simulink library "SUB_ECU_L4_MABX_HW_Interface_PTC_1571"  (R2018a)
settings: Solver=VariableStepAuto  StartTime=0.0  StopTime=10.0  RelTol=1e-3
PostLoadFcn:
  | , if any(exist('dsrtsu_mdlpostloadfcn', 'file') == [2, 3, 6]), try dsrtsu_mdlpostloadfcn('Execute', bdroot); catch fprintf('Error in PostLoadFcn (dsrtsu_mdlpostloadfcn) for model "%s":\n %s\n', bdroot, lasterr); end, end,
undefined symbols (not defined in the file or in its folder): CANR_PROPB_REAX_3_13_CHANNEL_APV, CANR_PROPB_REAX_4_13_CHANNEL_APV, CANR_PROPB_XPR_1_50_CHANNEL_APV, ENUM_CAN_RX_T, ENUM_CAN_TX_T, ENUM_REAX_OPERATION_MODE_T, ENUM_SIGNAL_HEALTH_T, ENUM_XBR_CONTROL_MODE_T, ENUM_XBR_EBI_MODE_T, ENUM_XBR_PASS_THROUGH_ACTIVE_T, ENUM_XBR_PRIORITY_T, ENUM_XPR_INHIBIT_PARK_MANUAL_T, ENUM_XPR_INHIBIT_UNPARK_MANUAL_T, ENUM_XPR_PARK_MANUAL_T, ENUM_XPR_UNPARK_MANUAL_T, IGNITION_RELAY_OVERRIDE_APV, INVERTER_RELAY_OVERRIDE_APV, MABX_RELAY_OVERRIDE_APV, PROPB_REAX_1_E4_DES_POS_SIG_SRC_APV, PROPB_REAX_1_E4_DESIRED_OPMODE_APV, PROPB_REAX_1_E4_DESIRED_POSITION_APV, ptc_matlab_lib, SENSOR_RELAY_OVERRIDE_APV, sfi, sfp
libraries: PTC_MBDS_LIB x163, rtican x81, simulink x41, EmE_MBD_Blockset x35, rti1401lib_dio_type4 x8, simulink_need_slupdate x7, $bdroot x5, rti1401lib_adc_type4 x2, rti1401lib_aio_type1 x1, rtitasklib x1
(part 4 of 27)

== system SUB_ECU_L4_MABX_HW_Interface_PTC_1571/OUTPUTS_PTC_1571 ==
  Outputs : Inport
  In : Inport  Port=2
  CAN_Out_PTC_1571 : $bdroot/CAN_Out_PTC_1571
  DIGITAL_out : $bdroot/DIGITAL_out
  wires:
  In/1 -> DIGITAL_out/2, CAN_Out_PTC_1571/2
  Outputs/1 -> DIGITAL_out/1, CAN_Out_PTC_1571/1

== system SUB_ECU_L4_MABX_HW_Interface_PTC_1571/CAN_Out_PTC_1571/CAN_TX_10000ms ==
  10000msCAN : Inport
  Terminator : Terminator
  wires:
  10000msCAN/1 -> Terminator/1

== system SUB_ECU_L4_MABX_HW_Interface_PTC_1571/CAN_Out_PTC_1571/CAN_TX_1000ms ==
  1000msCAN : Inport
  CAN_TX_AIR1_31 : Subsystem
  CAN_TX_AMB_00 : Subsystem
  Constant1 : Constant  Value=ENUM_CAN_TX_T.TX_CAN_4
  Constant2 : Constant  Value=ENUM_CAN_TX_T.TX_CAN_4
  wires:
  Constant1/1 -> CAN_TX_AMB_00/1(Channel)
  1000msCAN/1 -> CAN_TX_AIR1_31/2(Data), CAN_TX_AMB_00/2(Data)
  Constant2/1 -> CAN_TX_AIR1_31/1(Channel)

== system SUB_ECU_L4_MABX_HW_Interface_PTC_1571/CAN_Out_PTC_1571/CAN_TX_100ms ==
  100msCAN : Inport
  Feedthrough : Inport  Port=2
  Bus Selector : BusSelector  OutputSignals=INPUTS.DIO_Bus.OperatorEnableSwitch,INPUTS.CAN.VI_00.F_Truck166_VIN_Match
  Bus Selector1 : BusSelector  OutputSignals=INPUTS.DIO_Bus.OperatorEnableSwitch
  Bus Selector2 : BusSelector  OutputSignals=INPUTS.DIO_Bus.OperatorEnableSwitch,INPUTS.CAN.VI_00.F_Truck1571_VIN_Match
  CANT_PROPB_XPR_5B_CHANNEL_APV : Constant  Value=ENUM_CAN_TX_T.TX_CAN_1
  CANT_PROPB_XPR_FC_CHANNEL_APV : Constant  Value=ENUM_CAN_TX_T.TX_CAN_4
  CAN_TX_CCVS1_00 : Subsystem
  CAN_TX_CCVS1_31 : Subsystem
  CAN_TX_EBC2_0B : Subsystem
  CAN_TX_ETC2_03 : Subsystem
  CAN_TX_PROPB_REAX_5_E4 : Subsystem
  CAN_TX_PROPB_XPR_5B : Subsystem
  CAN_TX_PROPB_XPR_FC : Subsystem
  COGSRapidUpdate : Subsystem
  EBC1_8B : Subsystem
  EffortsValue : Subsystem
  Encode_PropB_REAX_5 : Subsystem
  Encode_PropB_XPR_5B : Subsystem
  Encode_PropB_XPR_FC : Subsystem  SystemSampleTime=0.1
  Logical Operator : Logic  OutDataTypeStr=boolean
  Logical Operator1 : Logic  OutDataTypeStr=boolean
  POSRapidUpdate : Subsystem
  PROPB_XPR_INHIBIT_PARK_MANUAL_APV : Constant  Value=ENUM_XPR_INHIBIT_PARK_MANUAL_T.NO_OVERRIDE
  PROPB_XPR_INHIBIT_UNPARK_MANUAL_APV : Constant  Value=ENUM_XPR_INHIBIT_UNPARK_MANUAL_T.NO_OVERRIDE
  PROPB_XPR_PARK_MANUAL_APV : Constant  Value=ENUM_XPR_PARK_MANUAL_T.NO_OVERRIDE
  PROPB_XPR_UNPARK_MANUAL_APV : Constant  Value=ENUM_XPR_UNPARK_MANUAL_T.NO_OVERRIDE
  enableCOGSRapidUpdateTX : Constant  Value=boolean(1)
  enableEBC1_8B_TX : Constant  Value=boolean(1)
  enablePosRapidUpdateTX : Constant  Value=boolean(1)
  wires:
  Feedthrough/1 -> CAN_TX_PROPB_REAX_5_E4/1(enable), CAN_TX_CCVS1_00/1(Data), COGSRapidUpdate/2(Data), CAN_TX_CCVS1_31/1(Data), CAN_TX_ETC2_03/1(Data), CAN_TX_EBC2_0B/1(Data), EBC1_8B/2(Data)
  Logical Operator1/1 -> CAN_TX_PROPB_XPR_FC/1(Enable)
  Bus Selector2/2 -> Logical Operator1/2  "<F_Truck1571_VIN_Match>"
  Bus Selector2/1 -> Logical Operator1/1  "<OperatorEnableSwitch>"
  Bus Selector/2 -> Logical Operator/2  "<F_Truck166_VIN_Match>"
  Logical Operator/1 -> CAN_TX_PROPB_XPR_5B/1(Enable)
  Bus Selector/1 -> Logical Operator/1  "<OperatorEnableSwitch>"
  Encode_PropB_XPR_5B/1(Data) -> CAN_TX_PROPB_XPR_5B/3(RawData)
  CANT_PROPB_XPR_5B_CHANNEL_APV/1 -> CAN_TX_PROPB_XPR_5B/2(Channel)
  enableEBC1_8B_TX/1 -> EBC1_8B/1(Enable)
  Encode_PropB_REAX_5/1(Data) -> CAN_TX_PROPB_REAX_5_E4/2(RawData)
  EffortsValue/1(EffortsValue) -> Encode_PropB_REAX_5/1(EffortsValue)
  Bus Selector1/1 -> Encode_PropB_XPR_FC/5(F_MessageEnable)  "<OperatorEnableSwitch>"
  CANT_PROPB_XPR_FC_CHANNEL_APV/1 -> CAN_TX_PROPB_XPR_FC/2(Channel)
  Encode_PropB_XPR_FC/1(Data) -> CAN_TX_PROPB_XPR_FC/3(RawData)
  PROPB_XPR_INHIBIT_UNPARK_MANUAL_APV/1 -> Encode_PropB_XPR_5B/2(inhibit_unpark_manual), Encode_PropB_XPR_FC/2(inhibit_unpark_manual)
  PROPB_XPR_PARK_MANUAL_APV/1 -> Encode_PropB_XPR_5B/3(park_manual), Encode_PropB_XPR_FC/3(park_manual)
  PROPB_XPR_UNPARK_MANUAL_APV/1 -> Encode_PropB_XPR_5B/4(unpark_manual), Encode_PropB_XPR_FC/4(unpark_manual)
  PROPB_XPR_INHIBIT_PARK_MANUAL_APV/1 -> Encode_PropB_XPR_5B/1(inhibit_park_manual), Encode_PropB_XPR_FC/1(inhibit_park_manual)
  enableCOGSRapidUpdateTX/1 -> COGSRapidUpdate/1(Enable)
  enablePosRapidUpdateTX/1 -> POSRapidUpdate/1(Enable)
  100msCAN/1 -> Bus Selector/1, Bus Selector1/1, POSRapidUpdate/2(Data), Bus Selector2/1

== system SUB_ECU_L4_MABX_HW_Interface_PTC_1571/CAN_Out_PTC_1571/CAN_TX_10ms ==
  10msCAN : Inport
  In : Inport  Port=2
  CANT_ACCS_E4_CHANNEL_APV : Constant  Value=ENUM_CAN_TX_T.TX_CAN_4
  CANT_EEC1_00_CHANNEL_APV : Constant  Value=ENUM_CAN_TX_T.TX_CAN_4_5
  CANT_VDC2_0B_CHANNEL_APV : Constant  Value=ENUM_CAN_TX_T.TX_CAN_5
  CAN_TX_ACCS_E4 : Subsystem
  CAN_TX_EEC1_00 : Subsystem
  CAN_TX_PROPB_REAX_1_E4 : Subsystem
  CAN_TX_VDC2_0B : Subsystem
  Encode_PROPB_REAX_1 : Subsystem
  wires:
  In/1 -> CAN_TX_PROPB_REAX_1_E4/1(enable), CAN_TX_EEC1_00/2(Data)
  CANT_ACCS_E4_CHANNEL_APV/1 -> CAN_TX_ACCS_E4/1(Channel)
  CANT_EEC1_00_CHANNEL_APV/1 -> CAN_TX_EEC1_00/1(Channel)
  Encode_PROPB_REAX_1/1(Out1) -> CAN_TX_PROPB_REAX_1_E4/2(RawData)
  CANT_VDC2_0B_CHANNEL_APV/1 -> CAN_TX_VDC2_0B/1(Channel)
  10msCAN/1 -> CAN_TX_VDC2_0B/2(Data), CAN_TX_ACCS_E4/2(Data), Encode_PROPB_REAX_1/1(In1)

== system SUB_ECU_L4_MABX_HW_Interface_PTC_1571/CAN_Out_PTC_1571/CAN_TX_20ms ==
  20msCAN : Inport
  Bus Selector : BusSelector  OutputSignals=INPUTS.DIO_Bus.OperatorEnableSwitch
  CANT_PROPB_XBR_B3_CHANNEL_APV : Constant  Value=ENUM_CAN_TX_T.TX_DISABLED
  CANT_STD_ODOMETRY_CHANNEL_APV : Constant  Value=ENUM_CAN_TX_T.TX_CAN_6
  CAN_TX_PROPB_XBR_B3 : Subsystem
  CAN_TX_PropB_2C2_XPR_65 : Subsystem
  CAN_TX_STD_ODOMETRY : Subsystem
  Encode_PropB_2C2_XPR : Subsystem
  Encode_PropB_XBR_B3 : Subsystem
  wires:
  Bus Selector/1 -> CAN_TX_PROPB_XBR_B3/3(OperatorEnable)  "<OperatorEnableSwitch>"
  Encode_PropB_XBR_B3/1(Out) -> CAN_TX_PROPB_XBR_B3/2(Data)
  CANT_PROPB_XBR_B3_CHANNEL_APV/1 -> CAN_TX_PROPB_XBR_B3/1(Channel)
  CANT_STD_ODOMETRY_CHANNEL_APV/1 -> CAN_TX_STD_ODOMETRY/1(Channel)
  20msCAN/1 -> CAN_TX_STD_ODOMETRY/2(Data), Bus Selector/1, Encode_PropB_2C2_XPR/1(In), Encode_PropB_XBR_B3/1(In)
  Encode_PropB_2C2_XPR/2(Out) -> CAN_TX_PropB_2C2_XPR_65/2(RawData)
  Encode_PropB_2C2_XPR/1(F_2C2_Enable) -> CAN_TX_PropB_2C2_XPR_65/1(Enable)

== system SUB_ECU_L4_MABX_HW_Interface_PTC_1571/CAN_Out_PTC_1571/CAN_TX_250ms ==
  250msCAN : Inport
  Terminator : Terminator
  wires:
  250msCAN/1 -> Terminator/1

== system SUB_ECU_L4_MABX_HW_Interface_PTC_1571/CAN_Out_PTC_1571/CAN_TX_5000ms ==
  5000msCAN : Inport
  Bus Selector : BusSelector  OutputSignals=INPUTS.DIO_Bus.OperatorEnableSwitch
  CAN_TX_RQST_13_E4 : Subsystem
  Encode_RQST : Subsystem
  RQST_13_E4_PGN : Subsystem
  wires:
  Bus Selector/1 -> CAN_TX_RQST_13_E4/2(OperatorEnable)  "<OperatorEnableSwitch>"
  5000msCAN/1 -> Bus Selector/1
  Encode_RQST/1(Data) -> CAN_TX_RQST_13_E4/1(RawData)
  RQST_13_E4_PGN/1(PGN) -> Encode_RQST/1(PGN)

== system SUB_ECU_L4_MABX_HW_Interface_PTC_1571/CAN_Out_PTC_1571/CAN_TX_50ms ==
  50msCAN : Inport
  CAN_TX_CCVS1 : Subsystem
  CAN_TX_TC1_05 : Subsystem
  enable_CAN_TX_CCVS1_CAN3 : Constant  OutDataTypeStr=Inherit: Inherit via back propagation
  wires:
  enable_CAN_TX_CCVS1_CAN3/1 -> CAN_TX_CCVS1/2(enable)
  50msCAN/1 -> CAN_TX_CCVS1/1(In1), CAN_TX_TC1_05/1(In1)

== system SUB_ECU_L4_MABX_HW_Interface_PTC_1571/CAN_Out_PTC_1571/CAN_TX_BAM ==
  CM : Subsystem
  Chart : Stateflow chart  TreatAsAtomicUnit=on
  Constant1 : Constant  Value=2  OutDataTypeStr=uint8
  DataFrame1 : Subsystem
  DataFrame2 : Subsystem
  Multiport Switch : MultiPortSwitch  Inputs=2  DiagnosticForDefault=Warning
  TX_TPCM : Subsystem
  TX_TPDT : Subsystem
  Terminator{,1..4} (5 alike) : Terminator
  Unit Delay1 : UnitDelay  InitialCondition=1  SampleTime=-1
  Unit Delay2 : UnitDelay  SampleTime=-1
  Unit Delay3 : UnitDelay  SampleTime=-1
  wires:
  Chart/5(TPDT_ts_Prev) -> Terminator4/1
  Chart/4(TPCM_ts_Prev) -> Terminator3/1
  Unit Delay1/1 -> Multiport Switch/1
  Unit Delay3/1 -> TX_TPDT/1(Trigger)
  Unit Delay2/1 -> TX_TPCM/1(Trigger)
  TX_TPDT/1(TX_status) -> Terminator1/1
  Chart/1(State) -> Terminator/1
  TX_TPCM/1(TX_status) -> Terminator2/1
  Chart/6(TPDT_count) -> Unit Delay1/1
  Chart/3(enTPCM) -> Unit Delay2/1
  Multiport Switch/1 -> TX_TPDT/2(Data)
  Constant1/1 -> Chart/3(TPDT_total)
  CM/1(Out1) -> TX_TPCM/2(Data)
  DataFrame2/1(Out1) -> Multiport Switch/3
  Chart/2(enTPDT) -> Unit Delay3/1
  DataFrame1/1(Out1) -> Multiport Switch/2
  TX_TPCM/2(TX_time) -> Chart/1(TPCM_ts)
  TX_TPDT/2(TX_time) -> Chart/2(TPDT_ts)

== system SUB_ECU_L4_MABX_HW_Interface_PTC_1571/CAN_Out_PTC_1571/CAN_TX_VariableRate ==
  Feedthrough : Inport
  CAN_TX_Std_SystemTime_01 : Subsystem
  wires:
  Feedthrough/1 -> CAN_TX_Std_SystemTime_01/1(Feedthrough)

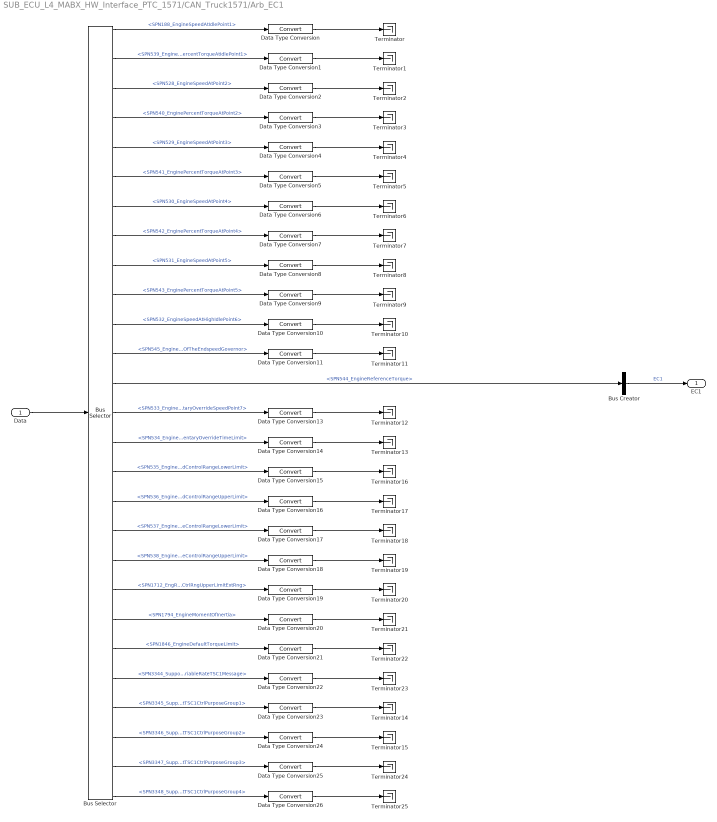
== system SUB_ECU_L4_MABX_HW_Interface_PTC_1571/CAN_Truck1571/Arb_EC1 ==
  Data : Inport
  Bus Creator : BusCreator  Inputs=1
  Bus Selector : BusSelector  OutputSignals=Signals.SPN188_EngineSpeedAtIdlePoint1,Signals.SPN539_EnginePercentTorqueAtIdlePoint1,Signals.SPN528_EngineSpeedAtPoint2,Signals.SPN540_EnginePercentTorqueAtPoint2,Signals.SPN529_EngineSpeedAtPoint3,Signals.SPN541_EnginePercentTorqueAtPoint3,Signals.SPN530_EngineSpeedAtPoint4,Signals.SPN542_EnginePercentTorqueAtPoint4,Signals.SPN531_EngineSpeedAtPoint5,Signals.SPN543_EnginePercentTorqueAtPoint5,Signals.SPN532_EngineSpeedAtHighIdlePoint6,Signals.SPN545_EngineGainKpOfTheEndspeedGovernor,Signals.SPN544_EngineReferenceTorque,Signals.SPN533_EngineMaximumMomentaryOverrideSpeedPoint7,Signals.SPN534_EngineMaximumMomentaryOverrideTimeLimit,Signals.SPN535_EngineRequestedSpeedControlRangeLowerLimit,Signals.SPN536_EngineRequestedSpeedControlRangeUpperLimit,Signals.SPN537_EngineRequestedTorqueControlRangeLowerLimit,Signals.SPN538_EngineRequestedTorqueControlRangeUpperLimit,Signals.SPN1712_EngRequestedSpeedCtrlRngUpperLimitExtRng,Signals.SPN1794_EngineMomentOfInertia,Signals.SPN1846_EngineDefaultTorqueLimit,Signals.SPN3344_SupportVariableRateTSC1Message,Signals.SPN3345_SupportTSC1CtrlPurposeGroup1,Signals.SPN3346_SupportTSC1CtrlPurposeGroup2,Signals.SPN3347_SupportTSC1CtrlPurposeGroup3,Signals.SPN3348_SupportTSC1CtrlPurposeGroup4
  Data Type Conversion{,1..11,13..26} (26 alike) : DataTypeConversion  SaturateOnIntegerOverflow=on
  Terminator{,1..25} (26 alike) : Terminator
      settings: InitFcn=|
      | try
      |    MBDS_BlockCallback('Update', gcb);
      | end
  EC1 : Outport
  wires:
  Data/1 -> Bus Selector/1
  Bus Selector/1 -> Data Type Conversion/1  "<SPN188_EngineSpeedAtIdlePoint1>"
  Bus Selector/12 -> Data Type Conversion11/1  "<SPN545_EngineGainKpOfTheEndspeedGovernor>"
  Bus Selector/2 -> Data Type Conversion1/1  "<SPN539_EnginePercentTorqueAtIdlePoint1>"
  Bus Selector/3 -> Data Type Conversion2/1  "<SPN528_EngineSpeedAtPoint2>"
  Bus Selector/4 -> Data Type Conversion3/1  "<SPN540_EnginePercentTorqueAtPoint2>"
  Bus Selector/5 -> Data Type Conversion4/1  "<SPN529_EngineSpeedAtPoint3>"
  Bus Selector/6 -> Data Type Conversion5/1  "<SPN541_EnginePercentTorqueAtPoint3>"
  Bus Selector/7 -> Data Type Conversion6/1  "<SPN530_EngineSpeedAtPoint4>"
  Bus Selector/8 -> Data Type Conversion7/1  "<SPN542_EnginePercentTorqueAtPoint4>"
  Bus Selector/9 -> Data Type Conversion8/1  "<SPN531_EngineSpeedAtPoint5>"
  Bus Selector/10 -> Data Type Conversion9/1  "<SPN543_EnginePercentTorqueAtPoint5>"
  Bus Selector/11 -> Data Type Conversion10/1  "<SPN532_EngineSpeedAtHighIdlePoint6>"
  Bus Selector/13 -> Bus Creator/1  "<SPN544_EngineReferenceTorque>"
  Bus Selector/14 -> Data Type Conversion13/1  "<SPN533_EngineMaximumMomentaryOverrideSpeedPoint7>"
  Bus Selector/15 -> Data Type Conversion14/1  "<SPN534_EngineMaximumMomentaryOverrideTimeLimit>"
  Bus Selector/16 -> Data Type Conversion15/1  "<SPN535_EngineRequestedSpeedControlRangeLowerLimit>"
  Bus Selector/17 -> Data Type Conversion16/1  "<SPN536_EngineRequestedSpeedControlRangeUpperLimit>"
  Bus Selector/18 -> Data Type Conversion17/1  "<SPN537_EngineRequestedTorqueControlRangeLowerLimit>"
  Bus Selector/19 -> Data Type Conversion18/1  "<SPN538_EngineRequestedTorqueControlRangeUpperLimit>"
  Bus Selector/20 -> Data Type Conversion19/1  "<SPN1712_EngRequestedSpeedCtrlRngUpperLimitExtRng>"
  Bus Selector/21 -> Data Type Conversion20/1  "<SPN1794_EngineMomentOfInertia>"
  Bus Selector/22 -> Data Type Conversion21/1  "<SPN1846_EngineDefaultTorqueLimit>"
  Bus Selector/23 -> Data Type Conversion22/1  "<SPN3344_SupportVariableRateTSC1Message>"
  Bus Selector/24 -> Data Type Conversion23/1  "<SPN3345_SupportTSC1CtrlPurposeGroup1>"
  Bus Selector/25 -> Data Type Conversion24/1  "<SPN3346_SupportTSC1CtrlPurposeGroup2>"
  Bus Selector/26 -> Data Type Conversion25/1  "<SPN3347_SupportTSC1CtrlPurposeGroup3>"
  Bus Selector/27 -> Data Type Conversion26/1  "<SPN3348_SupportTSC1CtrlPurposeGroup4>"
  Data Type Conversion/1 -> Terminator/1
  Data Type Conversion1/1 -> Terminator1/1
  Data Type Conversion2/1 -> Terminator2/1
  Data Type Conversion3/1 -> Terminator3/1
  Data Type Conversion6/1 -> Terminator6/1
  Data Type Conversion5/1 -> Terminator5/1
  Data Type Conversion7/1 -> Terminator7/1
  Data Type Conversion4/1 -> Terminator4/1
  Data Type Conversion9/1 -> Terminator9/1
  Data Type Conversion10/1 -> Terminator10/1
  Data Type Conversion13/1 -> Terminator12/1
  Data Type Conversion14/1 -> Terminator13/1
  Data Type Conversion15/1 -> Terminator16/1
  Data Type Conversion8/1 -> Terminator8/1
  Data Type Conversion11/1 -> Terminator11/1
  Data Type Conversion20/1 -> Terminator21/1
  Data Type Conversion22/1 -> Terminator23/1
  Data Type Conversion23/1 -> Terminator14/1
  Data Type Conversion17/1 -> Terminator18/1
  Data Type Conversion16/1 -> Terminator17/1
  Data Type Conversion21/1 -> Terminator22/1
  Data Type Conversion18/1 -> Terminator19/1
  Data Type Conversion19/1 -> Terminator20/1
  Data Type Conversion26/1 -> Terminator25/1
  Data Type Conversion25/1 -> Terminator24/1
  Data Type Conversion24/1 -> Terminator15/1
  Bus Creator/1 -> EC1/1  "EC1"

== system SUB_ECU_L4_MABX_HW_Interface_PTC_1571/CAN_Truck1571/Arb_PropB_REAX_3 ==
  Data : Inport
  Bus Selector : BusSelector  OutputSignals=Signals.PropB_REAX_3_CurrentOperatingMode,Signals.PropB_REAX_3_ReqOperatingMode,Signals.PropB_REAX_3_StatusErrMsg,Signals.PropB_REAX_3_HandwheelTorque,Signals.PropB_REAX_3_HandwheelVelocity,Signals.PropB_REAX_3_PullCompensation
  Data Type Conversion{,1..5} (6 alike) : DataTypeConversion  SaturateOnIntegerOverflow=on
  Terminator{,1..5} (6 alike) : Terminator
      settings: InitFcn=|
      | try
      |    MBDS_BlockCallback('Update', gcb);
      | end
  wires:
  Data/1 -> Bus Selector/1
  Bus Selector/2 -> Data Type Conversion1/1  "<PropB_REAX_3_ReqOperatingMode>"
  Bus Selector/4 -> Data Type Conversion3/1  "<PropB_REAX_3_HandwheelTorque>"
  Bus Selector/3 -> Data Type Conversion2/1  "<PropB_REAX_3_StatusErrMsg>"
  Bus Selector/1 -> Data Type Conversion/1  "<PropB_REAX_3_CurrentOperatingMode>"
  Bus Selector/5 -> Data Type Conversion4/1  "<PropB_REAX_3_HandwheelVelocity>"
  Bus Selector/6 -> Data Type Conversion5/1  "<PropB_REAX_3_PullCompensation>"
  Data Type Conversion/1 -> Terminator/1
  Data Type Conversion1/1 -> Terminator1/1
  Data Type Conversion2/1 -> Terminator2/1
  Data Type Conversion3/1 -> Terminator3/1
  Data Type Conversion4/1 -> Terminator4/1
  Data Type Conversion5/1 -> Terminator5/1

== system SUB_ECU_L4_MABX_HW_Interface_PTC_1571/CAN_Truck1571/Arb_PropB_REAX_4 ==
  Data : Inport
  Bus Selector : BusSelector  OutputSignals=Signals.PropB_REAX_4_AbsSteeringPosValid,Signals.PropB_REAX_4_PositionIndexValid,Signals.PropB_REAX_4_DriverControlledEffortsEnabled,Signals.PropB_REAX_4_ControlOperatingMode,Signals.PropB_REAX_4_SystemMode,Signals.PropB_REAX_4_PercHandwheelTorque,Signals.PropB_REAX_4_AbsSteeringAngle,Signals.PropB_REAX_4_PercMotorTorque
  Data Type Conversion{,1..7} (8 alike) : DataTypeConversion  SaturateOnIntegerOverflow=on
  Terminator{,1..7} (8 alike) : Terminator
      settings: InitFcn=|
      | try
      |    MBDS_BlockCallback('Update', gcb);
      | end
  wires:
  Data/1 -> Bus Selector/1
  Bus Selector/4 -> Data Type Conversion3/1  "<PropB_REAX_4_ControlOperatingMode>"
  Bus Selector/3 -> Data Type Conversion2/1  "<PropB_REAX_4_DriverControlledEffortsEnabled>"
  Bus Selector/5 -> Data Type Conversion4/1  "<PropB_REAX_4_SystemMode>"
  Bus Selector/2 -> Data Type Conversion/1  "<PropB_REAX_4_PositionIndexValid>"
  Bus Selector/1 -> Data Type Conversion1/1  "<PropB_REAX_4_AbsSteeringPosValid>"
  Bus Selector/6 -> Data Type Conversion5/1  "<PropB_REAX_4_PercHandwheelTorque>"
  Bus Selector/7 -> Data Type Conversion6/1  "<PropB_REAX_4_AbsSteeringAngle>"
  Bus Selector/8 -> Data Type Conversion7/1  "<PropB_REAX_4_PercMotorTorque>"
  Data Type Conversion1/1 -> Terminator/1
  Data Type Conversion/1 -> Terminator1/1
  Data Type Conversion2/1 -> Terminator2/1
  Data Type Conversion3/1 -> Terminator3/1
  Data Type Conversion4/1 -> Terminator4/1
  Data Type Conversion5/1 -> Terminator5/1
  Data Type Conversion6/1 -> Terminator6/1
  Data Type Conversion7/1 -> Terminator7/1

== system SUB_ECU_L4_MABX_HW_Interface_PTC_1571/CAN_Truck1571/CAN1_RX_TPCM_FF_00 ==
  Constant : Constant  Value=ENUM_CAN_RX_T.RX_CAN_1
  Multiport_Switch : MultiPortSwitch  DataPortOrder=Specify indices  DataPortIndices={ENUM_CAN_RX_T.RX_CAN_1, ENUM_CAN_RX_T.RX_CAN_2, ENUM_CAN_RX_T.RX_CAN_3, ENUM_CAN_RX_T.RX_CAN_4, ENUM_CAN_RX_T.RX_CAN_5, ENUM_CAN_RX_T.RX_CAN_6}  DataPortForDefault=Additional data port  SaturateOnIntegerOverflow=on  InputSameDT=on
      settings: AttributesFormatString=Zero-based indexing: %<zeroidx>
  RX_CAN_1 : Subsystem
  SelectChannel : Subsystem
  Terminator{,1..4} (5 alike) : Terminator
      settings: InitFcn=|
      | try
      |    MBDS_BlockCallback('Update', gcb);
      | end
  TPCM_FF_00 : Outport
  wires:
  Multiport_Switch/1 -> TPCM_FF_00/1
  SelectChannel/2(CAN2) -> Terminator/1
  SelectChannel/3(CAN3) -> Terminator1/1
  SelectChannel/4(CAN4) -> Terminator2/1
  SelectChannel/5(CAN5) -> Terminator3/1
  SelectChannel/6(CAN6) -> Terminator4/1
  RX_CAN_1/1(TPCM_FF_00) -> Multiport_Switch/2, Multiport_Switch/3, Multiport_Switch/4, Multiport_Switch/5, Multiport_Switch/6, Multiport_Switch/7, Multiport_Switch/8
  SelectChannel/1(CAN1) -> RX_CAN_1/1(Enable)
  Constant/1 -> Multiport_Switch/1, SelectChannel/1(In1)

== system SUB_ECU_L4_MABX_HW_Interface_PTC_1571/CAN_Truck1571/CAN1_RX_TPDT_FF_00 ==
  Constant : Constant  Value=ENUM_CAN_RX_T.RX_CAN_1
  Multiport_Switch : MultiPortSwitch  DataPortOrder=Specify indices  DataPortIndices={ENUM_CAN_RX_T.RX_CAN_1, ENUM_CAN_RX_T.RX_CAN_2, ENUM_CAN_RX_T.RX_CAN_3, ENUM_CAN_RX_T.RX_CAN_4, ENUM_CAN_RX_T.RX_CAN_5, ENUM_CAN_RX_T.RX_CAN_6}  DataPortForDefault=Additional data port  SaturateOnIntegerOverflow=on  InputSameDT=on
      settings: AttributesFormatString=Zero-based indexing: %<zeroidx>
  RX_CAN_1 : Subsystem
  SelectChannel : Subsystem
  Terminator{,1..4} (5 alike) : Terminator
      settings: InitFcn=|
      | try
      |    MBDS_BlockCallback('Update', gcb);
      | end
  TPDT_FF_00 : Outport
  wires:
  Constant/1 -> SelectChannel/1(In1), Multiport_Switch/1
  SelectChannel/1(CAN1) -> RX_CAN_1/1(Enable)
  RX_CAN_1/1(TPDT_FF_00) -> Multiport_Switch/8, Multiport_Switch/7, Multiport_Switch/6, Multiport_Switch/5, Multiport_Switch/4, Multiport_Switch/3, Multiport_Switch/2
  SelectChannel/6(CAN6) -> Terminator4/1
  SelectChannel/5(CAN5) -> Terminator3/1
  SelectChannel/4(CAN4) -> Terminator2/1
  SelectChannel/3(CAN3) -> Terminator1/1
  SelectChannel/2(CAN2) -> Terminator/1
  Multiport_Switch/1 -> TPDT_FF_00/1

== system SUB_ECU_L4_MABX_HW_Interface_PTC_1571/CAN_Truck1571/CAN_RX_ACC1_2A ==
  Constant : Constant  Value=boolean(1)
  RX_CAN_1 : Subsystem
  ACC1_2A : Outport
  wires:
  Constant/1 -> RX_CAN_1/1(Enable)
  RX_CAN_1/1(ACC1_2A) -> ACC1_2A/1

== system SUB_ECU_L4_MABX_HW_Interface_PTC_1571/CAN_Truck1571/CAN_RX_AEBS1_2A ==
  Constant : Constant  Value=boolean(1)
  RX_CAN_1 : Subsystem
  AEBS1_2A : Outport
  wires:
  RX_CAN_1/1(AEBS1_2A) -> AEBS1_2A/1
  Constant/1 -> RX_CAN_1/1(Enable)

== system SUB_ECU_L4_MABX_HW_Interface_PTC_1571/CAN_Truck1571/CAN_RX_AIR1_31 ==
  Constant : Constant  Value=boolean(1)
  RX_CAN_1 : Subsystem
  AIR1_31 : Outport
  wires:
  Constant/1 -> RX_CAN_1/1(Enable)
  RX_CAN_1/1(AIR1_31) -> AIR1_31/1

== system SUB_ECU_L4_MABX_HW_Interface_PTC_1571/CAN_Truck1571/CAN_RX_AMB_00 ==
  Constant : Constant  Value=boolean(1)
  RX_CAN_1 : Subsystem
  AMB_00 : Outport
  wires:
  RX_CAN_1/1(AMB_00) -> AMB_00/1
  Constant/1 -> RX_CAN_1/1(Enable)

== system SUB_ECU_L4_MABX_HW_Interface_PTC_1571/CAN_Truck1571/CAN_RX_B2_31 ==
  Constant : Constant
  RX_CAN_1 : Subsystem
  B2_00 : Outport
  wires:
  Constant/1 -> RX_CAN_1/1(Enable)
  RX_CAN_1/1(B2_31) -> B2_00/1

== system SUB_ECU_L4_MABX_HW_Interface_PTC_1571/CAN_Truck1571/CAN_RX_Bendix_RADAR_Tracks ==
  Constant : Constant  Value=boolean(1)
  RX_CAN_3 : Subsystem
  Bendix_RADAR_Tracks : Outport
  wires:
  Constant/1 -> RX_CAN_3/1(Enable)
  RX_CAN_3/1(Bendix_RADAR_Tracks) -> Bendix_RADAR_Tracks/1

== system SUB_ECU_L4_MABX_HW_Interface_PTC_1571/CAN_Truck1571/CAN_RX_CCVS1_00 ==
  Constant : Constant  Value=boolean(1)
  RX_CAN_1 : Subsystem
  CCVS1_0 : Outport
  wires:
  RX_CAN_1/1(CCVS1_0) -> CCVS1_0/1
  Constant/1 -> RX_CAN_1/1(Enable)

== system SUB_ECU_L4_MABX_HW_Interface_PTC_1571/CAN_Truck1571/CAN_RX_CCVS1_31 ==
  Constant : Constant  Value=boolean(1)
  RX_CAN_1 : Subsystem
  CCVS1_31 : Outport
  wires:
  Constant/1 -> RX_CAN_1/1(Enable)
  RX_CAN_1/1(CCVS1_31_) -> CCVS1_31/1

== system SUB_ECU_L4_MABX_HW_Interface_PTC_1571/CAN_Truck1571/CAN_RX_COGSOGRapidUpdate_01 ==
  Constant : Constant
  RX_CAN_4 : Subsystem
  COGSOGRapidUpdate_01 : Outport
  wires:
  RX_CAN_4/1(COGSOGRapidUpdate_01) -> COGSOGRapidUpdate_01/1
  Constant/1 -> RX_CAN_4/1(Enable)

== system SUB_ECU_L4_MABX_HW_Interface_PTC_1571/CAN_Truck1571/CAN_RX_CVW_0B ==
  Constant : Constant  Value=boolean(1)
  RX_CAN_1 : Subsystem
  CVW_0B : Outport
  wires:
  RX_CAN_1/1(CVW_0B) -> CVW_0B/1
  Constant/1 -> RX_CAN_1/1(Enable)

== system SUB_ECU_L4_MABX_HW_Interface_PTC_1571/CAN_Truck1571/CAN_RX_EBC1_0B ==
  Constant1 : Constant  Value=boolean(1)
  RX_CAN_1_EBC1 : Subsystem
  EBC1_0B : Outport
  wires:
  RX_CAN_1_EBC1/1(EBC1_0B_) -> EBC1_0B/1
  Constant1/1 -> RX_CAN_1_EBC1/1(Enable)

== system SUB_ECU_L4_MABX_HW_Interface_PTC_1571/CAN_Truck1571/CAN_RX_EBC1_8B ==
  Constant1 : Constant  Value=boolean(1)
  RX_CAN_2_EBC1 : Subsystem
  EBC1_8B : Outport
  wires:
  Constant1/1 -> RX_CAN_2_EBC1/1(Enable)
  RX_CAN_2_EBC1/1(EBC1_8B) -> EBC1_8B/1

== system SUB_ECU_L4_MABX_HW_Interface_PTC_1571/CAN_Truck1571/CAN_RX_EBC2_0B ==
  Enable_RX_EBC2_0B : Constant  Value=boolean(1)
  RX_CAN_1 : Subsystem
  EBC2_0B : Outport
  wires:
  RX_CAN_1/1(EBC2_0B) -> EBC2_0B/1
  Enable_RX_EBC2_0B/1 -> RX_CAN_1/1(Enable)

== system SUB_ECU_L4_MABX_HW_Interface_PTC_1571/CAN_Truck1571/CAN_RX_EC1_00 ==
  TPCM_BAM_CAN1 : Inport
  TPDT_BAM_CAN1 : Inport  Port=2
  timeStamp : Inport  Port=3
  Bus Creator : BusCreator  Inputs=5
  Bus Selector13 : BusSelector  OutputSignals=RX_status
  Bus Selector5 : BusSelector  OutputSignals=Signals.TPCM_BAM.SPN2569_ParameterGroupNumber
  CAN_RX_EC1_00 : Subsystem  TreatAsAtomicUnit=on
  Constant2 : Constant  Value=uint32(hex2dec('FEE3'))
  Decode_EC1 : PTC_MBDS_LIB/J1939/Decoders/Decode_EC1  PTC_MBDS_BlockVersion=5.41  PTC_BlockType=PTC_MBDS_Decode_EC1
      settings: SourceProductName=PACCAR Technical Center MBDS Library
  EQ1 : PTC_MBDS_LIB/MBDS Standard Library/Basic Operations/Logic and Bit Operations/EQ  InputSameDT=on  PTC_MBDS_BlockVersion=5.41  PTC_BlockType=PTC_MBDS_EQ
      settings: SourceProductName=PACCAR Technical Center MBDS Library
  Logical Operator : Logic  AllPortsSameDT=off  OutDataTypeStr=boolean
  EC1_00 : Outport
  wires:
  Bus Selector13/1 -> Logical Operator/1  "<RX_status>"
  [TPDT_BAM_CAN1] -> Bus Selector13/1
  Bus Selector5/1 -> EQ1/1  "<SPN2569_ParameterGroupNumber>"
  [TPCM_BAM_CAN1] -> Bus Selector5/1
  EQ1/1 -> Logical Operator/2
  Constant2/1 -> EQ1/2
  TPCM_BAM_CAN1/1 -> [TPCM_BAM_CAN1]
  [TPCM_BAM_CAN1] -> CAN_RX_EC1_00/1(TPCM)
  [TPDT_BAM_CAN1] -> CAN_RX_EC1_00/2(TPDT)
  [RX_time] -> Bus Creator/4
  [Signals] -> Bus Creator/1
  [RX_status] -> Bus Creator/3
  [RawData] -> Bus Creator/2
  [RX_delta_time] -> Bus Creator/5
  TPDT_BAM_CAN1/1 -> [TPDT_BAM_CAN1]
  Bus Creator/1 -> EC1_00/1
  CAN_RX_EC1_00/1(RawData) -> [RawData], Decode_EC1/1
  CAN_RX_EC1_00/3(RX_time) -> [RX_time]
  CAN_RX_EC1_00/4(RX_delta_time) -> [RX_delta_time]
  CAN_RX_EC1_00/2(RX_status) -> [RX_status]
  Decode_EC1/1 -> [Signals]
  Logical Operator/1 -> CAN_RX_EC1_00/Enable
  timeStamp/1 -> CAN_RX_EC1_00/3(timeStamp)

== system SUB_ECU_L4_MABX_HW_Interface_PTC_1571/CAN_Truck1571/CAN_RX_EEC1_00 ==
  Enable_RX_EEC1_00 : Constant  Value=boolean(1)
  RX_CAN_1 : Subsystem
  EEC1_00 : Outport
  wires:
  RX_CAN_1/1(EEC1_00) -> EEC1_00/1
  Enable_RX_EEC1_00/1 -> RX_CAN_1/1(Enable)

== system SUB_ECU_L4_MABX_HW_Interface_PTC_1571/CAN_Truck1571/CAN_RX_EEC2_00 ==
  Enable_RX_EEC2_00 : Constant  Value=boolean(1)
  RX_CAN_2 : Subsystem
  EEC2_00 : Outport
  wires:
  Enable_RX_EEC2_00/1 -> RX_CAN_2/1(Enable)
  RX_CAN_2/1(EEC2_00) -> EEC2_00/1

== system SUB_ECU_L4_MABX_HW_Interface_PTC_1571/CAN_Truck1571/CAN_RX_EEC3_00 ==
  Enable_RX_EEC3_00 : Constant  Value=boolean(1)
  RX_CAN_1 : Subsystem
  EEC3_00 : Outport
  wires:
  RX_CAN_1/1(EEC3_00) -> EEC3_00/1
  Enable_RX_EEC3_00/1 -> RX_CAN_1/1(Enable)

== system SUB_ECU_L4_MABX_HW_Interface_PTC_1571/CAN_Truck1571/CAN_RX_ETC2_03 ==
  Enable_RX_ETC2_03 : Constant  Value=boolean(1)
  RX_CAN_1 : Subsystem
  ETC2_03 : Outport
  wires:
  RX_CAN_1/1(ETC2_03) -> ETC2_03/1
  Enable_RX_ETC2_03/1 -> RX_CAN_1/1(Enable)

== system SUB_ECU_L4_MABX_HW_Interface_PTC_1571/CAN_Truck1571/CAN_RX_GNSSDOPs_00 ==
  Constant : Constant
  RX_CAN_4 : Subsystem
  GNSSDOPs_00 : Outport
  wires:
  RX_CAN_4/1(GNSSDOPs_00) -> GNSSDOPs_00/1
  Constant/1 -> RX_CAN_4/1(Enable)

== system SUB_ECU_L4_MABX_HW_Interface_PTC_1571/CAN_Truck1571/CAN_RX_HRW_0B ==
  Enable_HRW_RX_0B : Constant  Value=boolean(1)
  RX_CAN_1 : Subsystem
  HRW_0B : Outport
  wires:
  Enable_HRW_RX_0B/1 -> RX_CAN_1/1(Enable)
  RX_CAN_1/1(HRW_0B_) -> HRW_0B/1

== system SUB_ECU_L4_MABX_HW_Interface_PTC_1571/CAN_Truck1571/CAN_RX_PROPB_REAX_2_13 ==
  In1 : Inport
  Bus Selector : BusSelector  OutputSignals=EnablePropB_ReAX_CAN2,EnablePropB_ReAX_CAN1
  RX_CAN_1 : Subsystem
  RX_CAN_2 : Subsystem
  Switch : Switch  Criteria=u2 ~= 0
  PROPB_REAX_2_13 : Outport
  wires:
  RX_CAN_2/1(PROPB_REAX_2_13) -> Switch/1
  In1/1 -> Bus Selector/1
  Bus Selector/1 -> Switch/2, RX_CAN_2/1(Enable)  "<EnablePropB_ReAX_CAN2>"
  Bus Selector/2 -> RX_CAN_1/1(Enable)  "<EnablePropB_ReAX_CAN1>"
  RX_CAN_1/1(PROPB_REAX_2_13) -> Switch/3
  Switch/1 -> PROPB_REAX_2_13/1

== system SUB_ECU_L4_MABX_HW_Interface_PTC_1571/CAN_Truck1571/CAN_RX_PROPB_REAX_3_13 ==
  Constant : Constant  Value=CANR_PROPB_REAX_3_13_CHANNEL_APV
  Multiport_Switch : MultiPortSwitch  DataPortOrder=Specify indices  DataPortIndices={ENUM_CAN_RX_T.RX_CAN_1, ENUM_CAN_RX_T.RX_CAN_2, ENUM_CAN_RX_T.RX_CAN_3, ENUM_CAN_RX_T.RX_CAN_4, ENUM_CAN_RX_T.RX_CAN_5, ENUM_CAN_RX_T.RX_CAN_6}  DataPortForDefault=Additional data port  SaturateOnIntegerOverflow=on  InputSameDT=on
      settings: AttributesFormatString=Zero-based indexing: %<zeroidx>
  RX_CAN_1 : Subsystem
  SelectChannel : Subsystem
  Terminator{,1..4} (5 alike) : Terminator
      settings: InitFcn=|
      | try
      |    MBDS_BlockCallback('Update', gcb);
      | end
  PROPB_REAX_3_13 : Outport
  wires:
  Multiport_Switch/1 -> PROPB_REAX_3_13/1
  SelectChannel/2(CAN2) -> Terminator/1
  SelectChannel/3(CAN3) -> Terminator1/1
  SelectChannel/4(CAN4) -> Terminator2/1
  SelectChannel/5(CAN5) -> Terminator3/1
  SelectChannel/6(CAN6) -> Terminator4/1
  SelectChannel/1(CAN1) -> RX_CAN_1/1(Enable)
  Constant/1 -> Multiport_Switch/1, SelectChannel/1(In1)
  RX_CAN_1/1(PROPB_REAX_3_13) -> Multiport_Switch/3, Multiport_Switch/4, Multiport_Switch/5, Multiport_Switch/6, Multiport_Switch/7, Multiport_Switch/8, Multiport_Switch/2

== system SUB_ECU_L4_MABX_HW_Interface_PTC_1571/CAN_Truck1571/CAN_RX_PROPB_REAX_4_13 ==
  Constant : Constant  Value=CANR_PROPB_REAX_4_13_CHANNEL_APV
  Multiport_Switch : MultiPortSwitch  DataPortOrder=Specify indices  DataPortIndices={ENUM_CAN_RX_T.RX_CAN_1, ENUM_CAN_RX_T.RX_CAN_2, ENUM_CAN_RX_T.RX_CAN_3, ENUM_CAN_RX_T.RX_CAN_4, ENUM_CAN_RX_T.RX_CAN_5, ENUM_CAN_RX_T.RX_CAN_6}  DataPortForDefault=Additional data port  SaturateOnIntegerOverflow=on  InputSameDT=on
      settings: AttributesFormatString=Zero-based indexing: %<zeroidx>
  RX_CAN_1 : Subsystem
  SelectChannel : Subsystem
  Terminator{,1..4} (5 alike) : Terminator
      settings: InitFcn=|
      | try
      |    MBDS_BlockCallback('Update', gcb);
      | end
  PROPB_REAX_4_13 : Outport
  wires:
  Constant/1 -> SelectChannel/1(In1), Multiport_Switch/1
  SelectChannel/1(CAN1) -> RX_CAN_1/1(Enable)
  SelectChannel/6(CAN6) -> Terminator4/1
  SelectChannel/5(CAN5) -> Terminator3/1
  SelectChannel/4(CAN4) -> Terminator2/1
  SelectChannel/3(CAN3) -> Terminator1/1
  SelectChannel/2(CAN2) -> Terminator/1
  Multiport_Switch/1 -> PROPB_REAX_4_13/1
  RX_CAN_1/1(PROPB_REAX_4_13) -> Multiport_Switch/3, Multiport_Switch/4, Multiport_Switch/5, Multiport_Switch/6, Multiport_Switch/7, Multiport_Switch/8, Multiport_Switch/2

== system SUB_ECU_L4_MABX_HW_Interface_PTC_1571/CAN_Truck1571/CAN_RX_PROPB_XPR_1_50 ==
  Constant : Constant  Value=CANR_PROPB_XPR_1_50_CHANNEL_APV
  Multiport_Switch : MultiPortSwitch  DataPortOrder=Specify indices  DataPortIndices={ENUM_CAN_RX_T.RX_CAN_1, ENUM_CAN_RX_T.RX_CAN_2, ENUM_CAN_RX_T.RX_CAN_3, ENUM_CAN_RX_T.RX_CAN_4, ENUM_CAN_RX_T.RX_CAN_5, ENUM_CAN_RX_T.RX_CAN_6}  DataPortForDefault=Additional data port  SaturateOnIntegerOverflow=on  InputSameDT=on
      settings: AttributesFormatString=Zero-based indexing: %<zeroidx>
  RX_CAN_1 : Subsystem
  SelectChannel : Subsystem
  Terminator{,1..4} (5 alike) : Terminator
      settings: InitFcn=|
      | try
      |    MBDS_BlockCallback('Update', gcb);
      | end
  PROPB_XPR_1 : Outport
  wires:
  Constant/1 -> SelectChannel/1(In1), Multiport_Switch/1
  SelectChannel/1(CAN1) -> RX_CAN_1/1(Enable)
  SelectChannel/6(CAN6) -> Terminator4/1
  SelectChannel/5(CAN5) -> Terminator3/1
  SelectChannel/4(CAN4) -> Terminator2/1
  SelectChannel/3(CAN3) -> Terminator1/1
  SelectChannel/2(CAN2) -> Terminator/1
  Multiport_Switch/1 -> PROPB_XPR_1/1
  RX_CAN_1/1(PROPB_XPR_1_50) -> Multiport_Switch/3, Multiport_Switch/4, Multiport_Switch/5, Multiport_Switch/6, Multiport_Switch/7, Multiport_Switch/8, Multiport_Switch/2

== system SUB_ECU_L4_MABX_HW_Interface_PTC_1571/CAN_Truck1571/CAN_RX_PX2 ==
  Constant : Constant  Value=boolean(1)
  RX_CAN_6 : Subsystem
  PX2_Lane : Outport
  wires:
  Constant/1 -> RX_CAN_6/1(Enable)
  RX_CAN_6/1(PX2_Lane_) -> PX2_Lane/1

== system SUB_ECU_L4_MABX_HW_Interface_PTC_1571/CAN_Truck1571/CAN_RX_PosRapidUpdate_01 ==
  In1 : Inport
  Constant : Constant
  RX_CAN_2 : Subsystem
  PosRapidUpdate_01 : Outport
  wires:
  RX_CAN_2/1(PosRapidUpdate_01) -> PosRapidUpdate_01/1
  Constant/1 -> RX_CAN_2/1(Enable)
  In1/1 -> RX_CAN_2/2(In)

== system SUB_ECU_L4_MABX_HW_Interface_PTC_1571/CAN_Truck1571/CAN_RX_Prop2C2_Status_30 ==
  Constant : Constant
  RX_CAN_2 : Subsystem
  Prop2C2_Status_30 : Outport
  wires:
  RX_CAN_2/1(Prop2C2_Status_30) -> Prop2C2_Status_30/1
  Constant/1 -> RX_CAN_2/1(Enable)

== system SUB_ECU_L4_MABX_HW_Interface_PTC_1571/CAN_Truck1571/CAN_RX_SSI2_03 ==
  Constant : Constant
  RX_CAN_1 : Subsystem
  SSI2_03 : Outport
  wires:
  RX_CAN_1/1(SSI2_03) -> SSI2_03/1
  Constant/1 -> RX_CAN_1/1(Enable)

== system SUB_ECU_L4_MABX_HW_Interface_PTC_1571/CAN_Truck1571/CAN_RX_STD_PROPB_PX2_1_E2 ==
  CAN_RX-Enable_PX2_MapLaneEgoLeft : Constant  Value=boolean(1)
  RX_CAN_6 : Subsystem
  PX2_MapLaneEgoLeft : Outport
  wires:
  RX_CAN_6/1(CAN_RX_PX2_MapLaneEgoLeft) -> PX2_MapLaneEgoLeft/1
  CAN_RX-Enable_PX2_MapLaneEgoLeft/1 -> RX_CAN_6/1(Enable)

== system SUB_ECU_L4_MABX_HW_Interface_PTC_1571/CAN_Truck1571/CAN_RX_STD_PROPB_PX2_1_E3 ==
  CAN_RX-Enable_PX2_MapLaneEgoLeft : Constant  Value=boolean(1)
  RX_CAN_6 : Subsystem
  PX2_MapLaneEgoRight : Outport
  wires:
  CAN_RX-Enable_PX2_MapLaneEgoLeft/1 -> RX_CAN_6/1(Enable)
  RX_CAN_6/1(CAN_RX_PX2_MapLaneEgoRight) -> PX2_MapLaneEgoRight/1

== system SUB_ECU_L4_MABX_HW_Interface_PTC_1571/CAN_Truck1571/CAN_RX_STD_PROPB_PX2_1_E5 ==
  Constant : Constant  Value=boolean(1)
  RX_CAN_6 : Subsystem
  STD_PROPB_PX2_1_E5 : Outport
  wires:
  RX_CAN_6/1(STD_PROPB_PX2_1_E5) -> STD_PROPB_PX2_1_E5/1
  Constant/1 -> RX_CAN_6/1(Enable)

== system SUB_ECU_L4_MABX_HW_Interface_PTC_1571/CAN_Truck1571/CAN_RX_SystemTime_01 ==
  Constant : Constant
  RX_CAN_4 : Subsystem
  SystemTime_00 : Outport
  wires:
  RX_CAN_4/1(SystemTime_00) -> SystemTime_00/1
  Constant/1 -> RX_CAN_4/1(Enable)

== system SUB_ECU_L4_MABX_HW_Interface_PTC_1571/CAN_Truck1571/CAN_RX_TC1_05 ==
  Constant : Constant  Value=boolean(1)
  RX_CAN_2 : Subsystem
  TC1_05 : Outport
  wires:
  Constant/1 -> RX_CAN_2/1(Enable)
  RX_CAN_2/1(TC1_05) -> TC1_05/1

== system SUB_ECU_L4_MABX_HW_Interface_PTC_1571/CAN_Truck1571/CAN_RX_VDC1_0B ==
  Constant : Constant  Value=boolean(1)
  RX_CAN_1 : Subsystem
  VDC1_0B : Outport
  wires:
  Constant/1 -> RX_CAN_1/1(Enable)
  RX_CAN_1/1(VDC1_0B) -> VDC1_0B/1

== system SUB_ECU_L4_MABX_HW_Interface_PTC_1571/CAN_Truck1571/CAN_RX_VDC2_0B ==
  Constant : Constant  Value=boolean(1)
  RX_CAN_1 : Subsystem
  VDC2_0B : Outport
  wires:
  RX_CAN_1/1(VDC2_0B) -> VDC2_0B/1
  Constant/1 -> RX_CAN_1/1(Enable)

== system SUB_ECU_L4_MABX_HW_Interface_PTC_1571/CAN_Truck1571/CAN_RX_VEP1_03 ==
  Constant : Constant
  RX_CAN_1 : Subsystem
  VEP1_03 : Outport
  wires:
  Constant/1 -> RX_CAN_1/1(Enable)
  RX_CAN_1/1(VEP1_03) -> VEP1_03/1

== system SUB_ECU_L4_MABX_HW_Interface_PTC_1571/CAN_Truck1571/CAN_RX_VI_00 ==
  TPCM_BAM_CAN1 : Inport
  TPDT_BAM_CAN1 : Inport  Port=2
  timeStamp : Inport  Port=3
  Bus Creator : BusCreator  Inputs=5
  Bus Selector13 : BusSelector  OutputSignals=RX_status
  Bus Selector5 : BusSelector  OutputSignals=Signals.TPCM_BAM.SPN2569_ParameterGroupNumber
  CAN_RX_VI_00 : Subsystem  TreatAsAtomicUnit=on
  Constant2 : Constant  Value=uint32(hex2dec('FEEC'))
  Decode_VI : Subsystem
  EQ1 : PTC_MBDS_LIB/MBDS Standard Library/Basic Operations/Logic and Bit Operations/EQ  InputSameDT=on  PTC_MBDS_BlockVersion=5.41  PTC_BlockType=PTC_MBDS_EQ
      settings: SourceProductName=PACCAR Technical Center MBDS Library
  Logical Operator : Logic  AllPortsSameDT=off  OutDataTypeStr=boolean
  VI_00 : Outport
  wires:
  timeStamp/1 -> CAN_RX_VI_00/3(timeStamp)
  Logical Operator/1 -> CAN_RX_VI_00/Enable
  Decode_VI/1(VI) -> [Signals]
  CAN_RX_VI_00/2(RX_status) -> [RX_status]
  CAN_RX_VI_00/4(RX_delta_time) -> [RX_delta_time]
  CAN_RX_VI_00/3(RX_time) -> [RX_time]
  CAN_RX_VI_00/1(RawData) -> Decode_VI/1(RawData), [RawData]
  Bus Creator/1 -> VI_00/1
  TPDT_BAM_CAN1/1 -> [TPDT_BAM_CAN1]
  [RX_delta_time] -> Bus Creator/5
  [RawData] -> Bus Creator/2
  [RX_status] -> Bus Creator/3
  [Signals] -> Bus Creator/1
  [RX_time] -> Bus Creator/4
  [TPDT_BAM_CAN1] -> CAN_RX_VI_00/2(TPDT)
  [TPCM_BAM_CAN1] -> CAN_RX_VI_00/1(TPCM)
  TPCM_BAM_CAN1/1 -> [TPCM_BAM_CAN1]
  Constant2/1 -> EQ1/2
  EQ1/1 -> Logical Operator/2
  [TPCM_BAM_CAN1] -> Bus Selector5/1
  Bus Selector5/1 -> EQ1/1  "<SPN2569_ParameterGroupNumber>"
  [TPDT_BAM_CAN1] -> Bus Selector13/1
  Bus Selector13/1 -> Logical Operator/1  "<RX_status>"

== system SUB_ECU_L4_MABX_HW_Interface_PTC_1571/CAN_Truck1571/CAN_enable ==
  In1 : Inport
  Bus Creator : BusCreator  Inputs=3
  Bus Selector : BusSelector  OutputSignals=VI_00.Signals.F_Truck1571_VIN_Match,VI_00.Signals.F_Truck166_VIN_Match
  If_Then_Else : EmE_MBD_Blockset/Signal Routing/If_Then_Else
      settings: SourceProductName=PACCAR EmE MBD Blockset
  Logical Operator : Logic  Operator=NOT  OutDataTypeStr=boolean
  Terminator : Terminator
  useGPSSA0 : Constant  Value=true
  useGPSSA00 : Constant  Value=false
  useReAX_CAN_Ch1 : Constant  Value=true
  Out1 : Outport
  wires:
  Bus Creator/1 -> Out1/1
  In1/1 -> Bus Selector/1
  Bus Selector/2 -> Terminator/1  "<F_Truck166_VIN_Match>"
  If_Then_Else/1 -> Bus Creator/3  "useGPS_SA00"
  Bus Selector/1 -> If_Then_Else/1  "<F_Truck1571_VIN_Match>"
  useGPSSA00/1 -> If_Then_Else/2
  useGPSSA0/1 -> If_Then_Else/3
  useReAX_CAN_Ch1/1 -> Logical Operator/1, Bus Creator/1  "EnablePropB_ReAX_CAN1"
  Logical Operator/1 -> Bus Creator/2  "EnablePropB_ReAX_CAN2"

== system SUB_ECU_L4_MABX_HW_Interface_PTC_1571/CAN_Truck1571/Decode_PropB_REAX_3 ==
  RawData : Inport  OutDataTypeStr=uint8  PortDimensions=8
  Bus Creator : BusCreator  Inputs=8
  Bus Selector : BusSelector  OutputSignals=byte1
  Bus Selector1 : BusSelector  OutputSignals=byte2
  Bus Selector2 : BusSelector  OutputSignals=byte3,byte4
  Bus Selector3 : BusSelector  OutputSignals=byte5,byte6
  Bus Selector4 : BusSelector  OutputSignals=byte7,byte8
  Demux : Demux  Outputs=8
  MergeBuses : PTC_MBDS_LIB/Extras/Signal Routing/MergeBuses  NumberOfBuses=5  NumberOfBusesPrev=5  PTC_MBDS_BlockVersion=5.41  PTC_BlockType=PTC_MBDS_MergeBuses  DummyParameter=4DEKh6e82v
      settings: SourceProductName=PACCAR Technical Center MBDS Library
  decode_byte1 : Subsystem
  decode_byte2 : Subsystem
  decode_byte3_byte4 : Subsystem
  decode_byte5_byte6 : Subsystem
  decode_byte7_byte8 : Subsystem
  PROPB_REAX_3 : Outport
  wires:
  RawData/1 -> Demux/1
  Demux/1 -> Bus Creator/1  "byte1"
  Demux/2 -> Bus Creator/2  "byte2"
  Demux/3 -> Bus Creator/3  "byte3"
  Demux/4 -> Bus Creator/4  "byte4"
  Demux/5 -> Bus Creator/5  "byte5"
  Demux/6 -> Bus Creator/6  "byte6"
  Demux/7 -> Bus Creator/7  "byte7"
  Demux/8 -> Bus Creator/8  "byte8"
  Bus Creator/1 -> [RawData]
  MergeBuses/1 -> PROPB_REAX_3/1  "Signals"
  decode_byte2/1(Out) -> MergeBuses/2
  decode_byte1/1(Out) -> MergeBuses/1
  decode_byte3_byte4/1(Out) -> MergeBuses/3
  decode_byte5_byte6/1(Out) -> MergeBuses/4
  decode_byte7_byte8/1(Out) -> MergeBuses/5
  [RawData] -> Bus Selector4/1, Bus Selector3/1, Bus Selector2/1, Bus Selector1/1, Bus Selector/1
  Bus Selector/1 -> decode_byte1/1(byte1)  "<byte1>"
  Bus Selector1/1 -> decode_byte2/1(byte2)  "<byte2>"
  Bus Selector2/1 -> decode_byte3_byte4/1(byte3)  "<byte3>"
  Bus Selector2/2 -> decode_byte3_byte4/2(byte4)  "<byte4>"
  Bus Selector3/1 -> decode_byte5_byte6/1(byte5)  "<byte5>"
  Bus Selector3/2 -> decode_byte5_byte6/2(byte6)  "<byte6>"
  Bus Selector4/1 -> decode_byte7_byte8/1(byte7)  "<byte7>"
  Bus Selector4/2 -> decode_byte7_byte8/2(byte8)  "<byte8>"

== system SUB_ECU_L4_MABX_HW_Interface_PTC_1571/CAN_Truck1571/Decode_PropB_REAX_4 ==
  RawData : Inport  OutDataTypeStr=uint8  PortDimensions=8
  Bus Creator : BusCreator  Inputs=8
  Bus Selector : BusSelector  OutputSignals=byte1
  Bus Selector1 : BusSelector  OutputSignals=byte2
  Bus Selector2 : BusSelector  OutputSignals=byte3
  Bus Selector3 : BusSelector  OutputSignals=byte5
  Bus Selector4 : BusSelector  OutputSignals=byte6,byte7
  Bus Selector5 : BusSelector  OutputSignals=byte8
  Demux : Demux  Outputs=8
  MergeBuses : PTC_MBDS_LIB/Extras/Signal Routing/MergeBuses  NumberOfBuses=6  NumberOfBusesPrev=6  PTC_MBDS_BlockVersion=5.41  PTC_BlockType=PTC_MBDS_MergeBuses  DummyParameter=gf146dpl2V
      settings: SourceProductName=PACCAR Technical Center MBDS Library
  decode_byte1 : Subsystem
  decode_byte2 : Subsystem
  decode_byte3 : Subsystem
  decode_byte5 : Subsystem
  decode_byte6_byte7 : Subsystem
  decode_byte8 : Subsystem
  PROPB_REAX_4 : Outport
  wires:
  [RawData] -> Bus Selector/1, Bus Selector1/1, Bus Selector2/1, Bus Selector3/1, Bus Selector5/1, Bus Selector4/1
  MergeBuses/1 -> PROPB_REAX_4/1  "Signals"
  Bus Creator/1 -> [RawData]
  Demux/8 -> Bus Creator/8  "byte8"
  Demux/7 -> Bus Creator/7  "byte7"
  Demux/6 -> Bus Creator/6  "byte6"
  Demux/5 -> Bus Creator/5  "byte5"
  Demux/4 -> Bus Creator/4  "byte4"
  Demux/3 -> Bus Creator/3  "byte3"
  Demux/2 -> Bus Creator/2  "byte2"
  Demux/1 -> Bus Creator/1  "byte1"
  RawData/1 -> Demux/1
  Bus Selector/1 -> decode_byte1/1(byte1)  "<byte1>"
  Bus Selector1/1 -> decode_byte2/1(byte2)  "<byte2>"
  Bus Selector2/1 -> decode_byte3/1(byte3)  "<byte3>"
  Bus Selector3/1 -> decode_byte5/1(byte5)  "<byte5>"
  Bus Selector4/1 -> decode_byte6_byte7/1(byte6)  "<byte6>"
  Bus Selector4/2 -> decode_byte6_byte7/2(byte7)  "<byte7>"
  Bus Selector5/1 -> decode_byte8/1(byte8)  "<byte8>"
  decode_byte1/1(Out) -> MergeBuses/1
  decode_byte2/1(Out) -> MergeBuses/2
  decode_byte3/1(Out) -> MergeBuses/3
  decode_byte5/1(Out) -> MergeBuses/4
  decode_byte8/1(Out) -> MergeBuses/6
  decode_byte6_byte7/1(Out) -> MergeBuses/5

== system SUB_ECU_L4_MABX_HW_Interface_PTC_1571/DIGITAL/PWM pedal input management ==
  Pedal_1_pwm_freq_raw_value : Inport
  Pedal_1_pwm_dc_raw_value : Inport  Port=2
  Pedal_2_pwm_freq_raw_value : Inport  Port=3
  Pedal_2_pwm_dc_raw_value : Inport  Port=4
  Arbitrate pedal position output : Subsystem
  Determine common angle : Subsystem
  Diagnose pedal input signals : Subsystem
  Fault arbitration : Subsystem
  PWM signal filtering conversion : Subsystem
  Synchronization check sensor 1 and 2 : Subsystem
  Pedal_pwm_position : Outport
  wires:
  Arbitrate pedal position output/1(Pedal_pwm_position) -> Pedal_pwm_position/1
  [Pedal_synch_data_F_Hard] -> Arbitrate pedal position output/2(Pedal_synch_data_F_Hard)
  [F_Pedal_pwm_sens_total_failure] -> Arbitrate pedal position output/1(F_Pedal_pwm_sens_total_failure)
  Arbitrate pedal position output/2(DEFAULT_VALUE) -> Determine common angle/6(DEFAULT_VALUE), Fault arbitration/3(DEFAULT_VALUE)
  PWM signal filtering conversion/1(Pedal_1_pwm_undefault) -> Synchronization check sensor 1 and 2/2(Pedal_1_pwm_undefault), Fault arbitration/2(Pedal_1_pwm_undefault)
  PWM signal filtering conversion/2(Pedal_2_pwm_undefault) -> Synchronization check sensor 1 and 2/3(Pedal_2_pwm_undefault), Fault arbitration/5(Pedal_2_pwm_undefault)
  Fault arbitration/2(Pedal_2_pwm_angle_arbitrated) -> Determine common angle/5(Pedal_2_pwm_angle_arbitrated)
  Fault arbitration/1(Pedal_1_pwm_angle_arbitrated) -> Determine common angle/4(Pedal_1_pwm_angle_arbitrated)
  Synchronization check sensor 1 and 2/1(F_Pedal_pwm_sync_fault) -> [F_Pedal_pwm_sync_fault]
  Determine common angle/1(Pedal_pwm_angle_common) -> Arbitrate pedal position output/3(Pedal_pwm_angle_common), Synchronization check sensor 1 and 2/1(Pedal_pwm_angle_common)
  Pedal_1_pwm_freq_raw_value/1 -> Diagnose pedal input signals/1(Pedal_1_pwm_freq_raw_value)
  Pedal_1_pwm_dc_raw_value/1 -> PWM signal filtering conversion/1(Pedal _1_pwm_dc_raw_value), Diagnose pedal input signals/2(Pedal_1_pwm_dc_raw_value)
  Pedal_2_pwm_freq_raw_value/1 -> Diagnose pedal input signals/3(Pedal_2_pwm_freq_raw_value)
  Pedal_2_pwm_dc_raw_value/1 -> Diagnose pedal input signals/4(Pedal_2_pwm_dc_raw_value), PWM signal filtering conversion/2(Pedal _2_pwm_dc_raw_value)
  [F_Pedal_pwm_sync_fault] -> Diagnose pedal input signals/5(F_Pedal_pwm_sync_fault)
  Diagnose pedal input signals/2(F_Pedal_pwm_sens_total_failure) -> Determine common angle/2(F_Pedal_pwm_sens_total_failure), [F_Pedal_pwm_sens_total_failure]
  Diagnose pedal input signals/4(Pedal_synch_data.F_Hard) -> [Pedal_synch_data_F_Hard]
  Diagnose pedal input signals/3(Pedal_2_pwm_health_state) -> Determine common angle/3(Pedal_2_pwm_health_state), Fault arbitration/4(Pedal_2_pwm_health_state)
  Diagnose pedal input signals/1(Pedal_1_pwm_health_state) -> Determine common angle/1(Pedal_1_pwm_health_state), Fault arbitration/1(Pedal_1_pwm_health_state)

== system SUB_ECU_L4_MABX_HW_Interface_PTC_1571/DIGITAL/RationalityCheck ==
  UndefaultStatus : Inport
  Chart : Stateflow chart  TreatAsAtomicUnit=on
  DiagPassed : Outport
  wires:
  UndefaultStatus/1 -> Chart/1(Input)
  Chart/1(DiagPassed) -> DiagPassed/1

== system SUB_ECU_L4_MABX_HW_Interface_PTC_1571/DIGITAL_out/DIO_TYPE4_BIT_OUT_CH_BL2 ==
  In : Inport
  S-Function1 : S-Function  FunctionName=rti_commonblock  Parameters=sfi(1), sfp(1)  SFunctionDeploymentMode=off  EnableBusSupport=off
  wires:
  In/1 -> S-Function1/1

== system SUB_ECU_L4_MABX_HW_Interface_PTC_1571/DIGITAL_out/DIO_TYPE4_BIT_OUT_CH_BL3 ==
  In : Inport
  S-Function1 : S-Function  FunctionName=rti_commonblock  Parameters=sfi(1), sfp(1)  SFunctionDeploymentMode=off  EnableBusSupport=off
  wires:
  In/1 -> S-Function1/1

== system SUB_ECU_L4_MABX_HW_Interface_PTC_1571/DIGITAL_out/DIO_TYPE4_BIT_OUT_CH_BL4 ==
  In : Inport
  S-Function1 : S-Function  FunctionName=rti_commonblock  Parameters=sfi(1), sfp(1)  SFunctionDeploymentMode=off  EnableBusSupport=off
  wires:
  In/1 -> S-Function1/1

== system SUB_ECU_L4_MABX_HW_Interface_PTC_1571/DIGITAL_out/DIO_TYPE4_BIT_OUT_CH_BL5 ==
  In : Inport
  S-Function1 : S-Function  FunctionName=rti_commonblock  Parameters=sfi(1), sfp(1)  SFunctionDeploymentMode=off  EnableBusSupport=off
  wires:
  In/1 -> S-Function1/1

== system SUB_ECU_L4_MABX_HW_Interface_PTC_1571/DIGITAL_out/DIO_TYPE4_BIT_OUT_CH_BL6 ==
  In : Inport
  S-Function1 : S-Function  FunctionName=rti_commonblock  Parameters=sfi(1), sfp(1)  SFunctionDeploymentMode=off  EnableBusSupport=off
  wires:
  In/1 -> S-Function1/1

== system SUB_ECU_L4_MABX_HW_Interface_PTC_1571/DIGITAL_out/Determine pedal PWM and duty cycle values ==
  APTC_arb_pedal_position : Inport
  In : Inport  Port=2
  1-D Lookup Table2 : Lookup_n-D  NumberOfTableDimensions=1  BreakpointsForDimension1=[0 100]  Table=[10 45]  ExtrapMethod=Clip  UseLastTableValue=on  InputSameDT=on
      settings: AttributesFormatString=|
      | X: %<BreakpointsForDimension1>
      | Y: %<Table>
  1-D Lookup Table3 : Lookup_n-D  NumberOfTableDimensions=1  BreakpointsForDimension1=[0 100]  Table=[20 90]  ExtrapMethod=Clip  UseLastTableValue=on  InputSameDT=on
      settings: AttributesFormatString=|
      | X: %<BreakpointsForDimension1>
      | Y: %<Table>
  APTC_PEDAL_A_PWM_FREQ_HZ_APV : Constant  Value=200
  APTC_PEDAL_B_PWM_FREQ_HZ_APV : Constant  Value=200
  Bus Selector1 : BusSelector  OutputSignals=INPUTS.DIO_Bus.OperatorEnableSwitch
  Bus Selector4 : BusSelector  OutputSignals=INPUTS.DIO_Bus.Pedal_1_pwm_dc_raw_value
  Bus Selector5 : BusSelector  OutputSignals=INPUTS.DIO_Bus.Pedal_2_pwm_dc_raw_value
  Bus Selector6 : BusSelector  OutputSignals=INPUTS.DIO_Bus.Pedal_1_pwm_freq_raw_value
  Bus Selector7 : BusSelector  OutputSignals=INPUTS.DIO_Bus.Pedal_2_pwm_freq_raw_value
  If_Then_Else{1..2,4..5} (4 alike) : EmE_MBD_Blockset/Signal Routing/If_Then_Else
      settings: SourceProductName=PACCAR EmE MBD Blockset
  Logical Operator : Logic  Operator=NOT  OutDataTypeStr=boolean
  APTC_PWM_pedalA_freq_out : Outport
  APTC_PWM_pedalA_DC_out : Outport  Port=2
  APTC_PWM_pedalB_freq_out : Outport  Port=3
  APTC_PWM_pedalB_DC_out : Outport  Port=4
  wires:
  Bus Selector1/1 -> Logical Operator/1  "<OperatorEnableSwitch>"
  APTC_PEDAL_A_PWM_FREQ_HZ_APV/1 -> If_Then_Else4/3
  APTC_PEDAL_B_PWM_FREQ_HZ_APV/1 -> If_Then_Else5/3
  Bus Selector6/1 -> If_Then_Else4/2  "<Pedal_1_pwm_freq_raw_value>"
  Bus Selector4/1 -> If_Then_Else1/2  "<Pedal_1_pwm_dc_raw_value>"
  Bus Selector7/1 -> If_Then_Else5/2  "<Pedal_2_pwm_freq_raw_value>"
  Logical Operator/1 -> If_Then_Else2/1, If_Then_Else4/1, If_Then_Else5/1, If_Then_Else1/1
  Bus Selector5/1 -> If_Then_Else2/2  "<Pedal_2_pwm_dc_raw_value>"
  1-D Lookup Table3/1 -> If_Then_Else2/3  "PedalPWMB_DC_out"
  1-D Lookup Table2/1 -> If_Then_Else1/3  "PedalPWMA_DC_out"
  In/1 -> Bus Selector1/1, Bus Selector4/1, Bus Selector6/1, Bus Selector7/1, Bus Selector5/1
  APTC_arb_pedal_position/1 -> 1-D Lookup Table2/1, 1-D Lookup Table3/1
  If_Then_Else1/1 -> APTC_PWM_pedalA_DC_out/1
  If_Then_Else2/1 -> APTC_PWM_pedalB_DC_out/1
  If_Then_Else4/1 -> APTC_PWM_pedalA_freq_out/1
  If_Then_Else5/1 -> APTC_PWM_pedalB_freq_out/1
